simulink model "Comp_Model"  (R2019b)
settings: Solver=FixedStepDiscrete  StartTime=0.0  StopTime=10.0  RelTol=1e-3  EnableMultiTasking=on
undefined symbols (not defined in the file): stripchar_TMATS
libraries: Lib_Turbo_Compressor_TMATS x1
settings Model: Creator=jwchapm2  LastModifiedBy=bhisma
settings DataIOCC: LimitDataPoints=on  SaveFormat=Array  ReturnWorkspaceOutputs=off
settings OptimizationCC: LifeSpan=inf
settings DebuggingCC: SFUnexpectedBacktrackingDiag=warning  SFNoUnconditionalDefaultTransitionDiag=warning  SFExecutionAtInitializationDiag=none  ArithmeticOperatorsInVariantConditions=warning
settings HardwareCC: ProdBitPerPointer=32  ProdBitPerSizeT=32  ProdBitPerPtrDiffT=32  ProdLargestAtomicFloat=None  ProdIntDivRoundTo=Undefined  ProdEndianess=Unspecified  ProdWordSize=32  ProdHWDeviceType=32-bit Generic
settings ModelReferenceCC: PropagateSignalLabelsOutOfModel=off
settings SFSimCC: SimUseLocalCustomCode=off  CustomCodeUndefinedFunction=UseInterfaceOnly
settings RTWCC: RTWUseLocalCustomCode=off
settings CodeAppCC: StateflowObjectComments=on
settings GRTTargetCC: TargetLangStandard=C89/C90 (ANSI)  GeneratePreprocessorConditionals=Disable all
settings ConfigComp: CovMetricSettings=dw  CovHtmlReporting=on  CovSaveCumulativeToWorkspaceVar=on  CovSaveSingleToWorkspaceVar=on  CovExternalEMLEnable=off

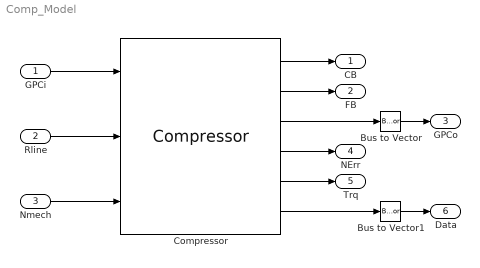
== system Comp_Model ==
  GPCi : Inport
  Rline : Inport  Port=2
  Nmech : Inport  Port=3
  Bus to Vector : BusToVector
  Bus to Vector1 : BusToVector
  Compressor : Lib_Turbo_Compressor_TMATS/Compressor  X_C_RlineVec_M=MWS.Comp.RlineVec  Z_C_AlphaVec_M=1  Y_C_Map_NcVec_M=MWS.Comp.NcVec  T_C_Map_WcArray_M=MWS.Comp.WcArray  T_C_Map_PRArray_M=MWS.Comp.PRArray  T_C_Map_EffArray_M=MWS.Comp.EffArray  s_C_Nc_M=MWS.Comp.s_Nc  s_C_Wc_M=MWS.Comp.s_Wc  s_C_PR_M=MWS.Comp.s_PR  s_C_Eff_M=MWS.Comp.s_eff  SL_M=off  Scale_M=none  CBLDEN_M=on  C_CBD_M=MWS.Comp.CBD  C_CBFht_M=MWS.Comp.CBFht  C_CBFPt_M=MWS.Comp.CBFPt  FBLDEN_M=on  C_FBD_M=MWS.Comp.FBD  C_BFht_M=MWS.Comp.FBht  C_BFPt_M=MWS.Comp.FBPt  DefSMEn_M=off  SRline_M=1  X_C_Map_WcSurgeVec_M=MWS.Comp.WcSurgeVec  T_C_Map_PRSurgeVec_M=MWS.Comp.PRSugeVec  iDesign_M=2  NcDes_M=10000  EffDes_M=0.95  PRDes_M=20  RlineDes_M=2  FVar_M=strcat('iDes_',stripchar_TMATS(gcb),'.bin')  BlkNm_M=double(gcb)  HP_M=off
  CB : Outport
  FB : Outport  Port=2
  GPCo : Outport  Port=3
  NErr : Outport  Port=4
  Trq : Outport  Port=5
  Data : Outport  Port=6
  wires:
  GPCi/1 -> Compressor/1
  Rline/1 -> Compressor/2
  Nmech/1 -> Compressor/3
  Compressor/1 -> CB/1
  Compressor/2 -> FB/1
  Compressor/6 -> Bus to Vector1/1
  Compressor/5 -> Trq/1
  Compressor/4 -> NErr/1
  Compressor/3 -> Bus to Vector/1
  Bus to Vector/1 -> GPCo/1
  Bus to Vector1/1 -> Data/1
